simulink model "TAK_01"  (R2023a)
settings: Solver=VariableStepAuto  StartTime=0.0  StopTime=40  MaxStep=0.01  RelTol=1e-3
settings Model: Creator=TDI  LastModifiedBy=TDI

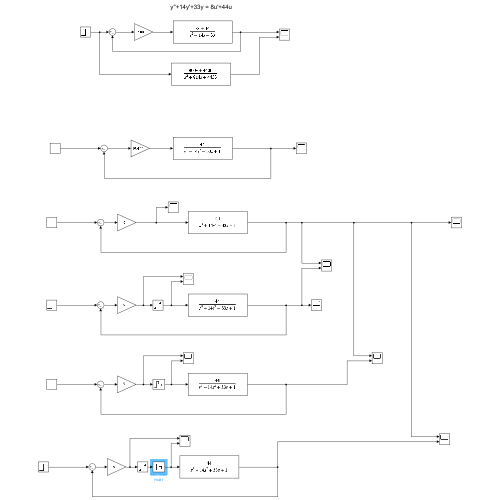
[thumbnail: Simulink's stored preview of the top-level diagram]
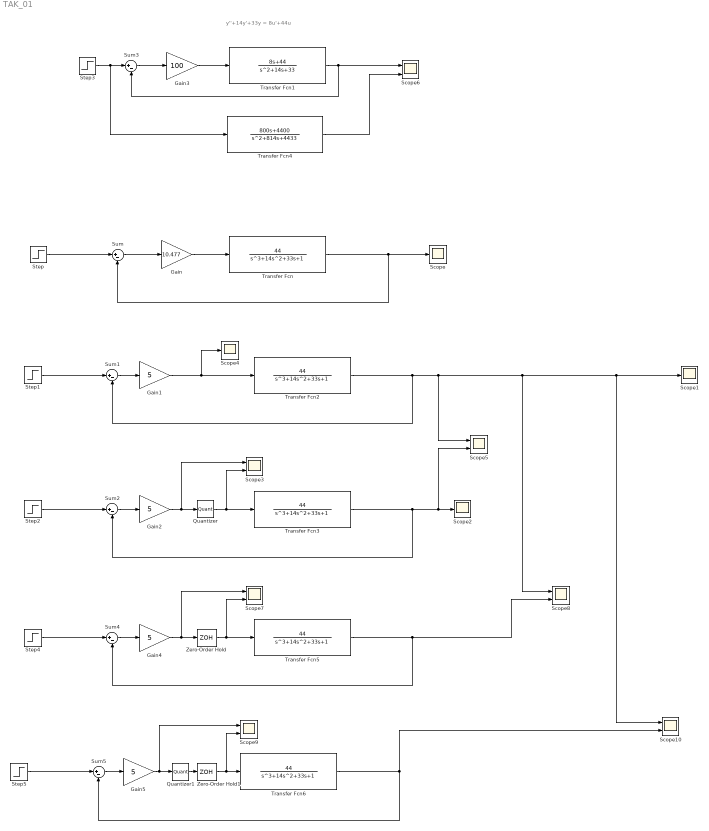
== system TAK_01 ==
  note: y''+14y'+33y = 8u'+44u
  Gain : Gain  Gain=10.477
  Gain{1..2,4..5} (4 alike) : Gain  Gain=5
  Gain3 : Gain  Gain=100
  Quantizer : Quantizer  QuantizationInterval=0.2
  Quantizer1 : Quantizer  QuantizationInterval=0.002
  Scope{,1..2,4} (4 alike) : Scope
  Scope{3,5..10} (7 alike) : Scope  NumInputPorts=2
  Step{,1..5} (6 alike) : Step  Time=0  SampleTime=0
  Sum{,1..5} (6 alike) : Sum  Inputs=|+-
  Transfer Fcn{,2..3,5..6} (5 alike) : TransferFcn  Numerator=[44]  Denominator=[1 14 33 1]
  Transfer Fcn1 : TransferFcn  Numerator=[8 44]  Denominator=[1 14 33]
  Transfer Fcn4 : TransferFcn  Numerator=[800 4400]  Denominator=[1 814 4433]
  Zero-Order Hold : ZeroOrderHold  SampleTime=0.1667
  Zero-Order Hold1 : ZeroOrderHold  SampleTime=0.004
  wires:
  Gain/1 -> Transfer Fcn/1
  Sum/1 -> Gain/1
  Step/1 -> Sum/1
  Transfer Fcn/1 -> Sum/2, Scope/1
  Step1/1 -> Sum1/1
  Gain1/1 -> Scope4/1, Transfer Fcn2/1
  Sum1/1 -> Gain1/1
  Transfer Fcn2/1 -> Sum1/2, Scope5/1, Scope8/1, Scope10/1, Scope1/1
  Sum2/1 -> Gain2/1
  Step2/1 -> Sum2/1
  Transfer Fcn3/1 -> Scope5/2, Scope2/1, Sum2/2
  Quantizer/1 -> Scope3/2, Transfer Fcn3/1
  Gain2/1 -> Scope3/1, Quantizer/1
  Sum3/1 -> Gain3/1
  Gain3/1 -> Transfer Fcn1/1
  Step3/1 -> Transfer Fcn4/1, Sum3/1
  Transfer Fcn1/1 -> Scope6/1, Sum3/2
  Transfer Fcn4/1 -> Scope6/2
  Gain4/1 -> Zero-Order Hold/1, Scope7/1
  Zero-Order Hold/1 -> Scope7/2, Transfer Fcn5/1
  Transfer Fcn5/1 -> Scope8/2, Sum4/2
  Sum4/1 -> Gain4/1
  Step4/1 -> Sum4/1
  Gain5/1 -> Quantizer1/1, Scope9/1
  Transfer Fcn6/1 -> Scope10/2, Sum5/2
  Sum5/1 -> Gain5/1
  Step5/1 -> Sum5/1
  Quantizer1/1 -> Zero-Order Hold1/1
  Zero-Order Hold1/1 -> Scope9/2, Transfer Fcn6/1
